simulink model "simple_model1"  (R2024a)
settings: Solver=VariableStepAuto  StartTime=0.0  StopTime=10.0  RelTol=1e-3
libraries: simulink x1
settings Model: Creator=tyang  LastModifiedBy=tyang

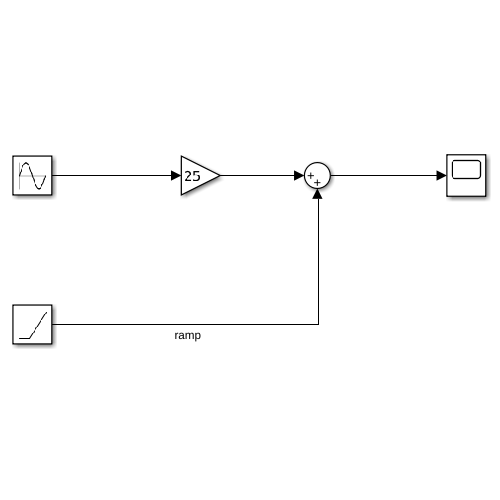
[thumbnail: Simulink's stored preview of the top-level diagram]
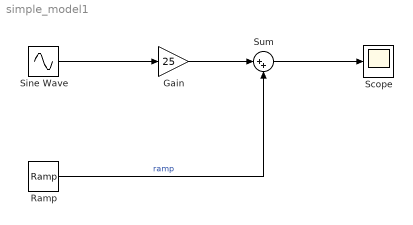
== system simple_model1 ==
  Gain : Gain  Gain=25
  Ramp : simulink/Sources/Ramp  slope=7  start=3  InitialOutput=0
  Scope : Scope
  Sine Wave : Sin  Amplitude=7  Frequency=8  SampleTime=0
  Sum : Sum  Inputs=|++
  wires:
  Sine Wave/1 -> Gain/1
  Gain/1 -> Sum/1
  Ramp/1 -> Sum/2  "ramp"
  Sum/1 -> Scope/1
